simulink model "polytopic_LPV"  (R2020a)
settings: Solver=ode15s  StartTime=0.0  StopTime=10.0  RelTol=1e-3  EnableMultiTasking=on
values from neighbouring files (symbols this model uses):
  p1max = 1/v_min    (= 0.166666666667)    [IPA_polytopes.m]
  p1min = 1/v_max    (= 0.025)    [IPA_polytopes.m]
  p2max = 1/(v_min.*v_min)    [IPA_polytopes.m]
  p2min = 1/(v_max.*v_max)    [IPA_polytopes.m]
  p3max = cos(d_min)    [IPA_polytopes.m]
  p3min = cos(d_max)    [IPA_polytopes.m]
undefined symbols (not defined in the file or in its folder): listK, sigbuilder_block
libraries: cstblocks x19, simulink x2
settings Model: Creator=AHMED  LastModifiedBy=lenovo ideapad
settings DataIOCC: LimitDataPoints=on  SaveFormat=Array  ReturnWorkspaceOutputs=off
settings OptimizationCC: LifeSpan=inf
settings DebuggingCC: SolverPrmCheckMsg=warning  SFUnexpectedBacktrackingDiag=warning  SFNoUnconditionalDefaultTransitionDiag=warning  SFExecutionAtInitializationDiag=none  ArithmeticOperatorsInVariantConditions=warning
settings HardwareCC: ProdBitPerPointer=32  ProdBitPerSizeT=32  ProdBitPerPtrDiffT=32  ProdLargestAtomicFloat=None  ProdIntDivRoundTo=Undefined  ProdEndianess=Unspecified  ProdWordSize=32  ProdHWDeviceType=32-bit Generic
settings ModelReferenceCC: PropagateSignalLabelsOutOfModel=off
settings SFSimCC: SimUseLocalCustomCode=off  CustomCodeUndefinedFunction=UseInterfaceOnly
settings RTWCC: RTWUseLocalCustomCode=off
settings CodeAppCC: StateflowObjectComments=on
settings GRTTargetCC: TargetLangStandard=C89/C90 (ANSI)
settings ConfigComp: CovMetricSettings=dw  CovHtmlReporting=on  CovSaveCumulativeToWorkspaceVar=on  CovSaveSingleToWorkspaceVar=on  CovExternalEMLEnable=off  CovSFcnEnable=off

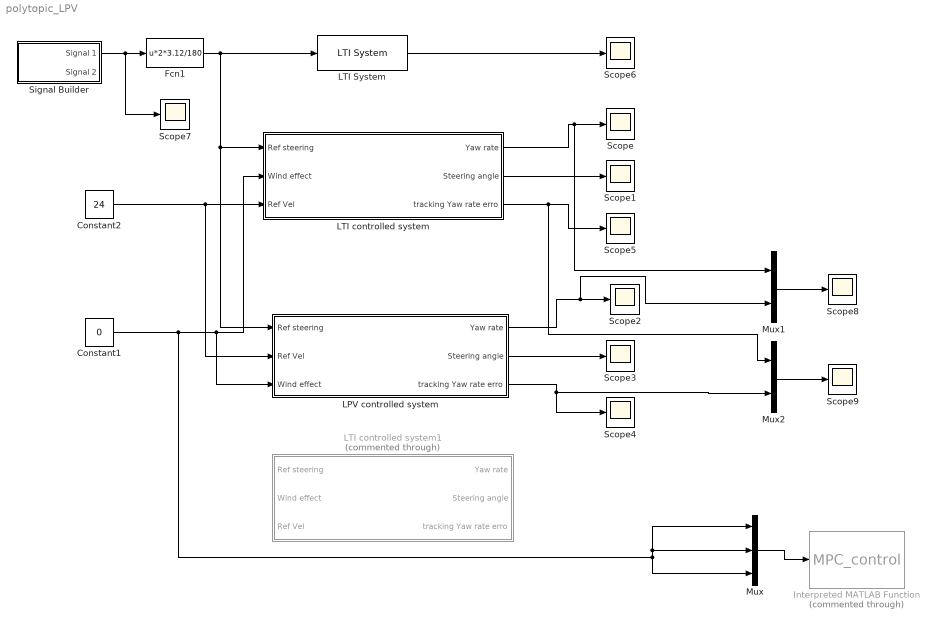
== system polytopic_LPV ==
  Constant1 : Constant  Value=0
  Constant2 : Constant  Value=24
  Fcn1 : Fcn  Expr=u*2*3.12/180
  Interpreted MATLAB Function : MATLABFcn  Commented=through  MATLABFcn=MPC_control  OutputDimensions=3
  LPV controlled system : Subsystem
  LTI System : cstblocks/LTI System  sys=Pr  IC=[]
  LTI controlled system : Subsystem
  LTI controlled system1 : Subsystem  Commented=through
  Mux : Mux  Inputs=3
  Mux1 : Mux  Inputs=2
  Mux2 : Mux  Inputs=2
  Scope{,1..9} (10 alike) : Scope
  Signal Builder : Subsystem  Tag=STV Subsys  LoadFcn=sigbuilder_block('load');  StartFcn=sigbuilder_block('start');  StopFcn=sigbuilder_block('stop');  ClipboardFcn=sigbuilder_block('clipboard');  mask(Sigbuilder block){tuvar=[0:10]}
      mask help: Simulink:masks:SigbuilderBlock_MD
      mask init:
      | if ~strcmp(get_param(bdroot(gcbh),'SimulationStatus'),'stopped') tuvar = sigbuilder_block('maskInit'); end
      settings: CopyFcn=sigbuilder_block('copy');  DeleteFcn=sigbuilder_block('delete');  ModelCloseFcn=sigbuilder_block('modelClose');  PreSaveFcn=sigbuilder_block('preSave');  PauseFcn=sigbuilder_block('pause');  ContinueFcn=sigbuilder_block('continue');  NameChangeFcn=sigbuilder_block('namechange');  OpenFcn=sigbuilder_block('open',[6 28.5 1012.5 483.75 ]);  CloseFcn=sigbuilder_block('close');
      mask Display: plot(0, 0, 100, 100,[2, 2, 32, 32, 2], [68, 8, 8, 68, 68],[32, 2], [38, 38], [32, 19, 2],[53, 60, 44], [32, 17, 17, 2],[16, 16, 31, 31]);txt = getActiveGroup(gcbh);text(2, 100, txt,'verticalAlignment', 'top');
  wires:
  LTI controlled system/1(Yaw rate) -> Mux1/1, Scope/1
  LTI controlled system/2(Steering angle) -> Scope1/1
  LPV controlled system/1(Yaw rate) -> Mux1/2, Scope2/1
  LPV controlled system/2(Steering angle) -> Scope3/1
  Constant2/1 -> LPV controlled system/2(Ref Vel), LTI controlled system/3(Ref Vel)
  Constant1/1 -> Mux/2, Mux/1, Mux/3, LPV controlled system/3(Wind effect), LTI controlled system/2(Wind effect)
  Fcn1/1 -> LTI System/1, LPV controlled system/1(Ref steering), LTI controlled system/1(Ref steering)
  LTI System/1 -> Scope6/1
  Mux/1 -> Interpreted MATLAB Function/1
  Signal Builder/1(Signal 1) -> Scope7/1, Fcn1/1
  Mux1/1 -> Scope8/1
  LTI controlled system/3(tracking Yaw rate erro) -> Mux2/1, Scope5/1
  LPV controlled system/3(tracking Yaw rate erro) -> Mux2/2, Scope4/1
  Mux2/1 -> Scope9/1

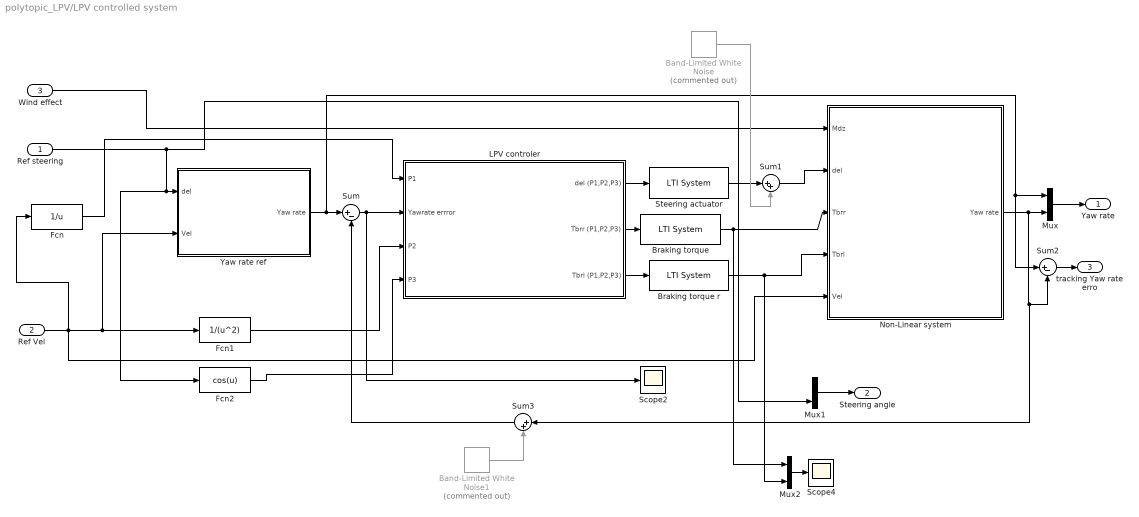
== system polytopic_LPV/LPV controlled system ==
  Ref steering : Inport
  Ref Vel : Inport  Port=2
  Wind effect : Inport  Port=3
  Band-Limited White Noise : simulink/Sources/Band-Limited White Noise  Commented=on  Cov=[0.1]  Ts=0.1  seed=[23341]
  Band-Limited White Noise1 : simulink/Sources/Band-Limited White Noise  Commented=on  Cov=[0.1]  Ts=0.1  seed=[23341]
  Braking torque : cstblocks/LTI System  sys=WactBr  IC=[]
  Braking torque r : cstblocks/LTI System  sys=WactBl  IC=[]
  Fcn : Fcn  Expr=1/u
  Fcn1 : Fcn  Expr=1/(u^2)
  Fcn2 : Fcn  Expr=cos(u)
  LPV controler : Subsystem
  Mux : Mux  Inputs=2
  Mux1 : Mux  Inputs=2
  Mux2 : Mux  Inputs=2
  Non-Linear system : Subsystem
  Scope2 : Scope
  Scope4 : Scope
  Steering actuator : cstblocks/LTI System  sys=WactS  IC=[]
  Sum : Sum  Inputs=|+-
  Sum1 : Sum  Inputs=|++
  Sum2 : Sum  Inputs=|+-
  Sum3 : Sum  Inputs=|++
  Yaw rate ref : Subsystem
  Yaw rate : Outport
  Steering angle : Outport  Port=2
  tracking Yaw rate erro : Outport  Port=3
  wires:
  Sum/1 -> LPV controler/2("Yawrate errror "), Scope2/1
  Wind effect/1 -> Non-Linear system/1(Mdz)
  Ref Vel/1 -> Non-Linear system/5(Vel), Yaw rate ref/2(Vel), Fcn1/1, Fcn/1
  Ref steering/1 -> Mux1/2, Yaw rate ref/1(del), Fcn2/1
  Mux/1 -> Yaw rate/1
  Mux2/1 -> Scope4/1
  Mux1/1 -> Steering angle/1
  Fcn2/1 -> LPV controler/4(P3)
  LPV controler/1(del (P1,P2,P3)) -> Steering actuator/1
  LPV controler/3(Tbrl (P1,P2,P3)) -> Braking torque r/1
  LPV controler/2(Tbrr (P1,P2,P3)) -> Braking torque/1
  Fcn/1 -> LPV controler/1(P1)
  Fcn1/1 -> LPV controler/3(P2)
  Yaw rate ref/1(Yaw rate) -> Sum/1, Sum2/1, Mux/1
  Non-Linear system/1(Yaw rate) -> Sum3/1, Sum2/2, Mux/2
  Sum2/1 -> tracking Yaw rate erro/1
  Braking torque/1 -> Mux2/1, Non-Linear system/3(Tbrr)
  Braking torque r/1 -> Mux2/2, Non-Linear system/4(Tbrl)
  Steering actuator/1 -> Sum1/1
  Band-Limited White Noise/1 -> Sum1/2
  Sum1/1 -> Non-Linear system/2(del)
  Sum3/1 -> Sum/2
  Band-Limited White Noise1/1 -> Sum3/2

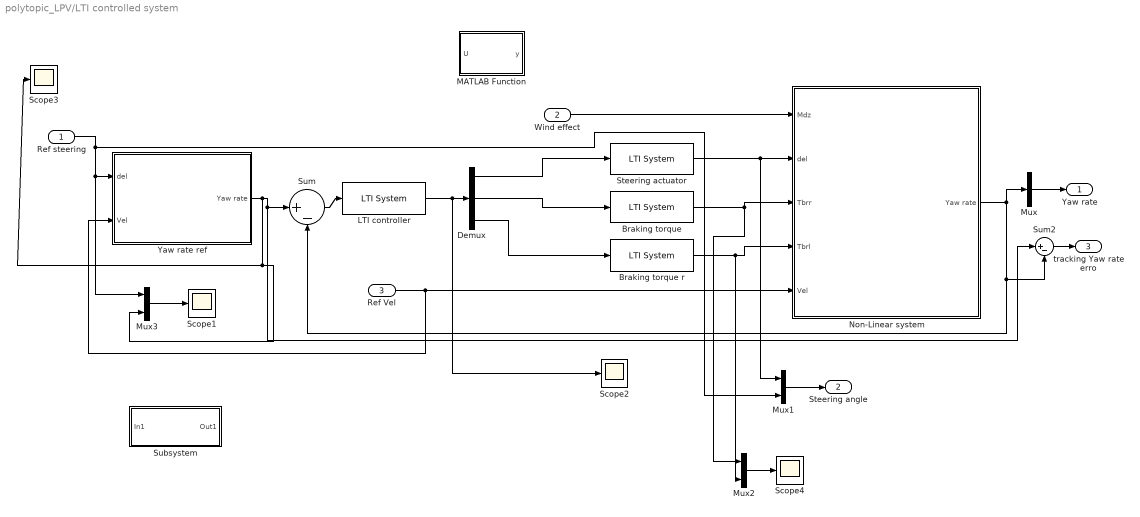
== system polytopic_LPV/LTI controlled system ==
  Ref steering : Inport
  Wind effect : Inport  Port=2
  Ref Vel : Inport  Port=3
  Braking torque : cstblocks/LTI System  sys=WactBr  IC=[]
  Braking torque r : cstblocks/LTI System  sys=WactBl  IC=[]
  Demux : Demux  Outputs=3
  LTI controller : cstblocks/LTI System  sys=KLTI  IC=[]
  MATLAB Function : MATLAB Function  TreatAsAtomicUnit=on
  Mux : Mux  Inputs=1
  Mux1 : Mux  Inputs=2
  Mux2 : Mux  Inputs=2
  Mux3 : Mux  Inputs=2
  Non-Linear system : Subsystem
  Scope{1..4} (4 alike) : Scope
  Steering actuator : cstblocks/LTI System  sys=WactS  IC=[]
  Subsystem : Subsystem
  Sum : Sum  Inputs=|+-
  Sum2 : Sum  Inputs=|+-
  Yaw rate ref : Subsystem
  Yaw rate : Outport
  Steering angle : Outport  Port=2
  tracking Yaw rate erro : Outport  Port=3
  wires:
  Yaw rate ref/1(Yaw rate) -> Sum2/1, Sum/1, Mux3/2, Scope3/1
  Sum/1 -> LTI controller/1
  LTI controller/1 -> Scope2/1, Demux/1
  Non-Linear system/1(Yaw rate) -> Mux/1, Sum2/2, Sum/2
  Wind effect/1 -> Non-Linear system/1(Mdz)
  Ref Vel/1 -> Yaw rate ref/2(Vel), Non-Linear system/5(Vel)
  Ref steering/1 -> Mux1/2, Yaw rate ref/1(del), Mux3/1
  Mux/1 -> Yaw rate/1
  Demux/1 -> Steering actuator/1
  Braking torque r/1 -> Mux2/2, Non-Linear system/4(Tbrl)
  Demux/3 -> Braking torque r/1
  Steering actuator/1 -> Non-Linear system/2(del), Mux1/1
  Demux/2 -> Braking torque/1
  Braking torque/1 -> Mux2/1, Non-Linear system/3(Tbrr)
  Mux2/1 -> Scope4/1
  Mux1/1 -> Steering angle/1
  Mux3/1 -> Scope1/1
  Sum2/1 -> tracking Yaw rate erro/1

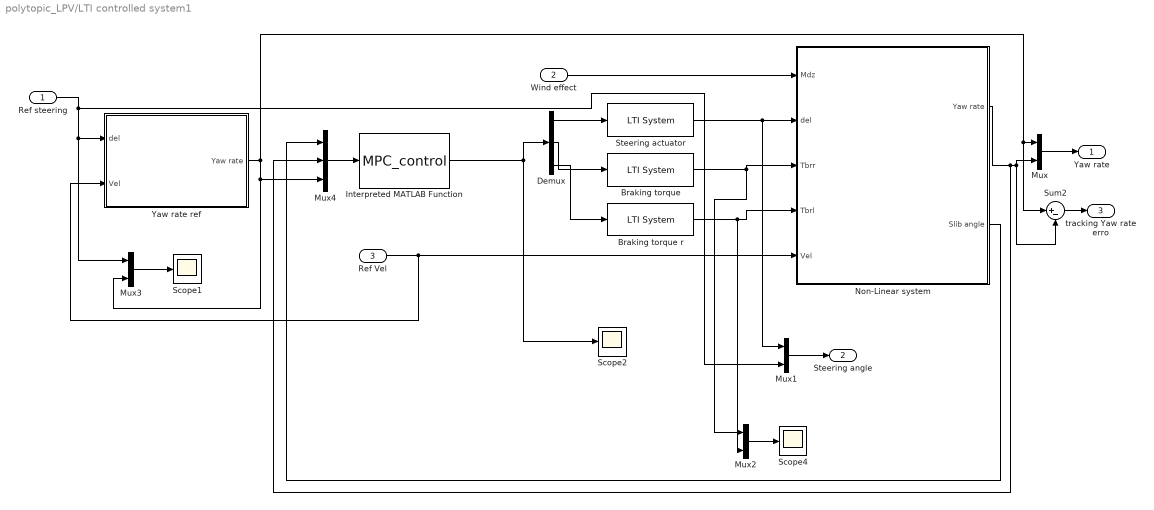
== system polytopic_LPV/LTI controlled system1 ==
  Ref steering : Inport
  Wind effect : Inport  Port=2
  Ref Vel : Inport  Port=3
  Braking torque : cstblocks/LTI System  sys=WactBr  IC=[]
  Braking torque r : cstblocks/LTI System  sys=WactBl  IC=[]
  Demux : Demux  Outputs=3
  Interpreted MATLAB Function : MATLABFcn  MATLABFcn=MPC_control  OutputDimensions=3
  Mux{,1..3} (4 alike) : Mux  Inputs=2
  Mux4 : Mux  Inputs=3
  Non-Linear system : Subsystem
  Scope1 : Scope
  Scope2 : Scope
  Scope4 : Scope
  Steering actuator : cstblocks/LTI System  sys=WactS  IC=[]
  Sum2 : Sum  Inputs=|+-
  Yaw rate ref : Subsystem
  Yaw rate : Outport
  Steering angle : Outport  Port=2
  tracking Yaw rate erro : Outport  Port=3
  wires:
  Yaw rate ref/1(Yaw rate) -> Mux4/3, Mux3/2, Sum2/1, Mux/1
  Interpreted MATLAB Function/1 -> Scope2/1, Demux/1
  Non-Linear system/1(Yaw rate) -> Mux4/2, Sum2/2, Mux/2
  Wind effect/1 -> Non-Linear system/1(Mdz)
  Ref Vel/1 -> Yaw rate ref/2(Vel), Non-Linear system/5(Vel)
  Ref steering/1 -> Mux1/2, Yaw rate ref/1(del), Mux3/1
  Mux/1 -> Yaw rate/1
  Demux/1 -> Steering actuator/1
  Braking torque r/1 -> Mux2/2, Non-Linear system/4(Tbrl)
  Demux/3 -> Braking torque r/1
  Steering actuator/1 -> Non-Linear system/2(del), Mux1/1
  Demux/2 -> Braking torque/1
  Braking torque/1 -> Mux2/1, Non-Linear system/3(Tbrr)
  Mux2/1 -> Scope4/1
  Mux1/1 -> Steering angle/1
  Mux3/1 -> Scope1/1
  Sum2/1 -> tracking Yaw rate erro/1
  Mux4/1 -> Interpreted MATLAB Function/1
  Non-Linear system/2(Slib angle) -> Mux4/1

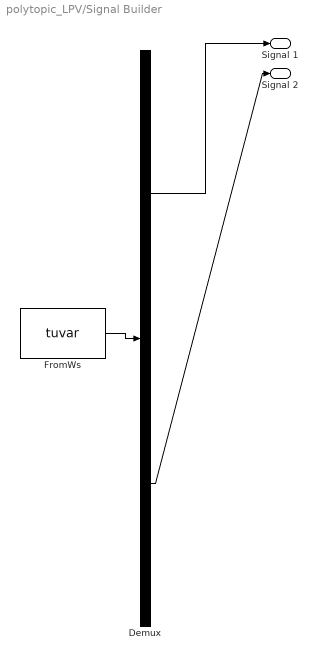
== system polytopic_LPV/Signal Builder ==
  Demux : Demux  Tag=STV Demux  Outputs=2
      settings: DisplayOption=none
  FromWs : FromWorkspace  Tag=STV FromWs  VariableName=tuvar
      SigBuilderData=|
      | common.afterFinalStr = 'Extrapolate'
      | common.sampleTime = 0
      | dataSet.timeRange = [0 10]
      | dataSet.name = 'Group 1'
      | sbobj.Groups.Name = 'Group 1'
      | sbobj.Groups.Signals(1).Name = 'Signal 1'
      | sbobj.Groups.Signals(1).XData = [0 0.98 2 2 3.02 3.02 4.96 4.96 6.04 6.04 6.98 10]
      | sbobj.Groups.Signals(1).YData = [0 0 10 9.95 9.95 10.05 -10 -10.05 -10.05 -9.9 -0.02 0]
      | sbobj.Groups.Signals(2).Name = 'Signal 2'
      | sbobj.Groups.Signals(2).XData = [0 2.04 2.04 2.58 2.58 4.94 4.94 6.98 10]
      | sbobj.Groups.Signals(2).YData = [0 0 0.01 11.2 11.3 11.3 11.4 0 0]
  Signal 1 : Outport  Tag=STV Outport
  Signal 2 : Outport  Tag=STV Outport  Port=2
  wires:
  Demux/1 -> Signal 1/1
  FromWs/1 -> Demux/1
  Demux/2 -> Signal 2/1

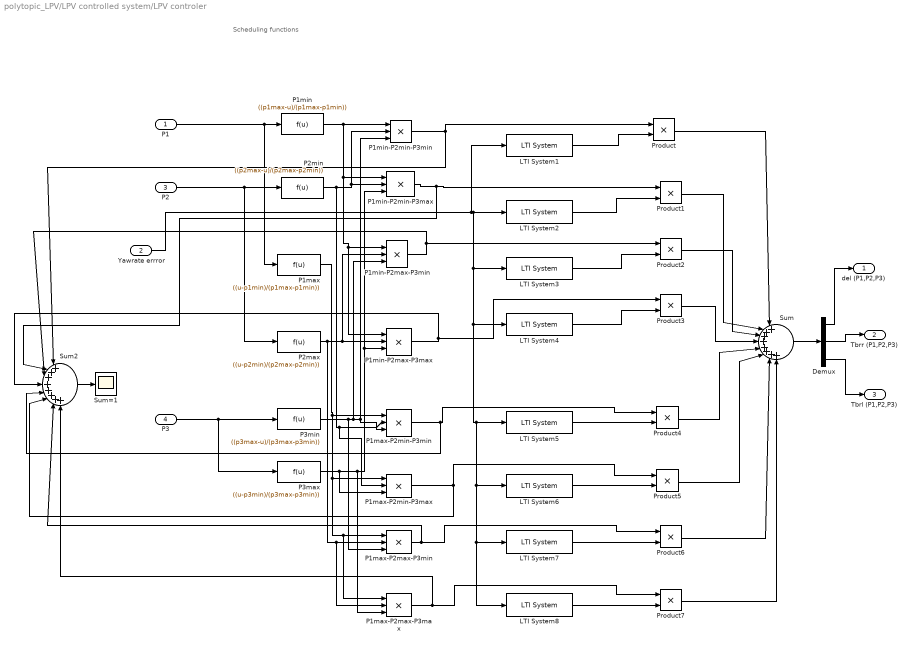
== system polytopic_LPV/LPV controlled system/LPV controler ==
  note: Scheduling functions
  P1 : Inport
  "Yawrate errror " : Inport  Port=2
  P2 : Inport  Port=3
  P3 : Inport  Port=4
  Demux : Demux  Outputs=3
  LTI System1 : cstblocks/LTI System  sys=listK{1}  IC=[]
  LTI System2 : cstblocks/LTI System  sys=listK{2}  IC=[]
  LTI System3 : cstblocks/LTI System  sys=listK{3}  IC=[]
  LTI System4 : cstblocks/LTI System  sys=listK{4}  IC=[]
  LTI System5 : cstblocks/LTI System  sys=listK{5}  IC=[]
  LTI System6 : cstblocks/LTI System  sys=listK{6}  IC=[]
  LTI System7 : cstblocks/LTI System  sys=listK{7}  IC=[]
  LTI System8 : cstblocks/LTI System  sys=listK{8}  IC=[]
  P1max : Fcn  Expr=((u-p1min)/(p1max-p1min))
  P1max-P2max-P3max : Product  Inputs=3
  P1max-P2max-P3min : Product  Inputs=3
  P1max-P2min-P3max : Product  Inputs=3
  P1max-P2min-P3min : Product  Inputs=3
  P1min : Fcn  Expr=((p1max-u)/(p1max-p1min))
  P1min-P2max-P3max : Product  Inputs=3
  P1min-P2max-P3min : Product  Inputs=3
  P1min-P2min-P3max : Product  Inputs=3
  P1min-P2min-P3min : Product  Inputs=3
  P2max : Fcn  Expr=((u-p2min)/(p2max-p2min))
  P2min : Fcn  Expr=((p2max-u)/(p2max-p2min))
  P3max : Fcn  Expr=((u-p3min)/(p3max-p3min))
  P3min : Fcn  Expr=((p3max-u)/(p3max-p3min))
  Product{,1..7} (8 alike) : Product
  Sum : Sum  Inputs=|++++++++
  Sum2 : Sum  Inputs=|++++++++
  Sum=1 : Scope
  del (P1,P2,P3) : Outport
  Tbrr (P1,P2,P3) : Outport  Port=2
  Tbrl (P1,P2,P3) : Outport  Port=3
  wires:
  "Yawrate errror "/1 -> LTI System1/1, LTI System8/1, LTI System7/1, LTI System6/1, LTI System5/1, LTI System4/1, LTI System3/1, LTI System2/1
  LTI System1/1 -> Product/2
  P1min-P2min-P3min/1 -> Product/1, Sum2/1
  P1min-P2min-P3max/1 -> Sum2/2, Product1/1
  LTI System2/1 -> Product1/2
  P1min-P2max-P3min/1 -> Product2/1, Sum2/3
  LTI System3/1 -> Product2/2
  P1min-P2max-P3max/1 -> Product3/1, Sum2/4
  LTI System4/1 -> Product3/2
  Product/1 -> Sum/1
  Product1/1 -> Sum/2
  Product2/1 -> Sum/3
  Product3/1 -> Sum/4
  P2max/1 -> P1max-P2max-P3max/2, P1max-P2max-P3min/2, P1min-P2max-P3min/2, P1min-P2max-P3max/2
  P2min/1 -> P1max-P2min-P3max/2, P1max-P2min-P3min/2, P1min-P2min-P3max/2, P1min-P2min-P3min/2
  P1min/1 -> P1min-P2max-P3max/1, P1min-P2max-P3min/1, P1min-P2min-P3max/1, P1min-P2min-P3min/1
  P1/1 -> P1max/1, P1min/1
  P2/1 -> P2max/1, P2min/1
  Sum2/1 -> Sum=1/1
  P3/1 -> P3max/1, P3min/1
  P3min/1 -> P1max-P2max-P3min/3, P1min-P2max-P3min/3, P1min-P2min-P3min/3, P1max-P2min-P3min/3
  P3max/1 -> P1max-P2min-P3max/3, P1min-P2min-P3max/3, P1min-P2max-P3max/3, P1max-P2max-P3max/3
  P1max/1 -> P1max-P2max-P3max/1, P1max-P2max-P3min/1, P1max-P2min-P3max/1, P1max-P2min-P3min/1
  LTI System5/1 -> Product4/2
  LTI System6/1 -> Product5/2
  LTI System7/1 -> Product6/2
  LTI System8/1 -> Product7/2
  P1max-P2min-P3min/1 -> Sum2/5, Product4/1
  P1max-P2min-P3max/1 -> Product5/1, Sum2/6
  P1max-P2max-P3min/1 -> Product6/1, Sum2/7
  P1max-P2max-P3max/1 -> Product7/1, Sum2/8
  Product4/1 -> Sum/5
  Product5/1 -> Sum/6
  Product6/1 -> Sum/7
  Product7/1 -> Sum/8
  Sum/1 -> Demux/1
  Demux/1 -> del (P1,P2,P3)/1
  Demux/2 -> Tbrr (P1,P2,P3)/1
  Demux/3 -> Tbrl (P1,P2,P3)/1

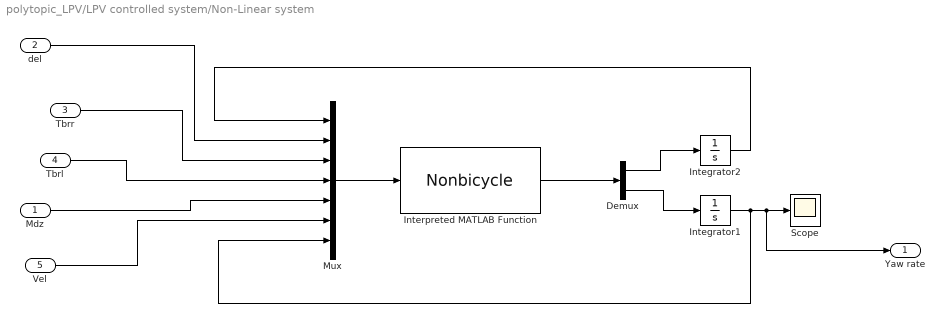
== system polytopic_LPV/LPV controlled system/Non-Linear system ==
  Mdz : Inport
  del : Inport  Port=2
  Tbrr : Inport  Port=3
  Tbrl : Inport  Port=4
  Vel : Inport  Port=5
  Demux : Demux  Outputs=2
  Integrator1 : Integrator
  Integrator2 : Integrator
  Interpreted MATLAB Function : MATLABFcn  MATLABFcn=Nonbicycle  OutputDimensions=2
  Mux : Mux  Inputs=7
  Scope : Scope
  Yaw rate : Outport
  wires:
  Mux/1 -> Interpreted MATLAB Function/1
  Interpreted MATLAB Function/1 -> Demux/1
  Demux/1 -> Integrator2/1
  Demux/2 -> Integrator1/1
  Integrator2/1 -> Mux/1
  Integrator1/1 -> Yaw rate/1, Scope/1, Mux/7
  del/1 -> Mux/2
  Vel/1 -> Mux/6
  Tbrr/1 -> Mux/3
  Tbrl/1 -> Mux/4
  Mdz/1 -> Mux/5

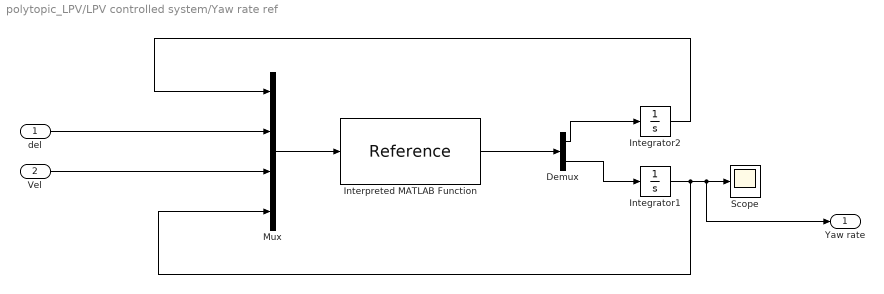
== system polytopic_LPV/LPV controlled system/Yaw rate ref ==
  del : Inport
  Vel : Inport  Port=2
  Demux : Demux  Outputs=2
  Integrator1 : Integrator
  Integrator2 : Integrator
  Interpreted MATLAB Function : MATLABFcn  MATLABFcn=Reference  OutputDimensions=2
  Mux : Mux
  Scope : Scope
  Yaw rate : Outport
  wires:
  Mux/1 -> Interpreted MATLAB Function/1
  Interpreted MATLAB Function/1 -> Demux/1
  Demux/1 -> Integrator2/1
  Demux/2 -> Integrator1/1
  Integrator2/1 -> Mux/1
  Integrator1/1 -> Mux/4, Yaw rate/1, Scope/1
  del/1 -> Mux/2
  Vel/1 -> Mux/3

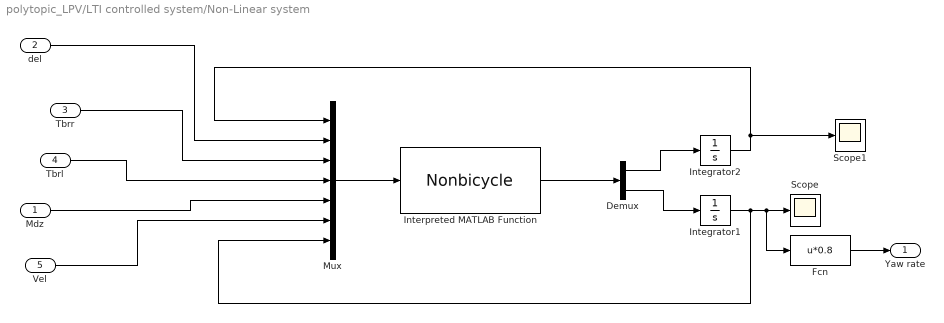
== system polytopic_LPV/LTI controlled system/Non-Linear system ==
  Mdz : Inport
  del : Inport  Port=2
  Tbrr : Inport  Port=3
  Tbrl : Inport  Port=4
  Vel : Inport  Port=5
  Demux : Demux  Outputs=2
  Fcn : Fcn  Expr=u*0.8
  Integrator1 : Integrator
  Integrator2 : Integrator
  Interpreted MATLAB Function : MATLABFcn  MATLABFcn=Nonbicycle  OutputDimensions=2
  Mux : Mux  Inputs=7
  Scope : Scope
  Scope1 : Scope
  Yaw rate : Outport
  wires:
  Mux/1 -> Interpreted MATLAB Function/1
  Interpreted MATLAB Function/1 -> Demux/1
  Demux/1 -> Integrator2/1
  Demux/2 -> Integrator1/1
  Integrator2/1 -> Scope1/1, Mux/1
  Integrator1/1 -> Fcn/1, Scope/1, Mux/7
  del/1 -> Mux/2
  Vel/1 -> Mux/6
  Tbrr/1 -> Mux/3
  Tbrl/1 -> Mux/4
  Mdz/1 -> Mux/5
  Fcn/1 -> Yaw rate/1

== system polytopic_LPV/LTI controlled system/Subsystem ==
  In1 : Inport
  Out1 : Outport
  wires:
  In1/1 -> Out1/1

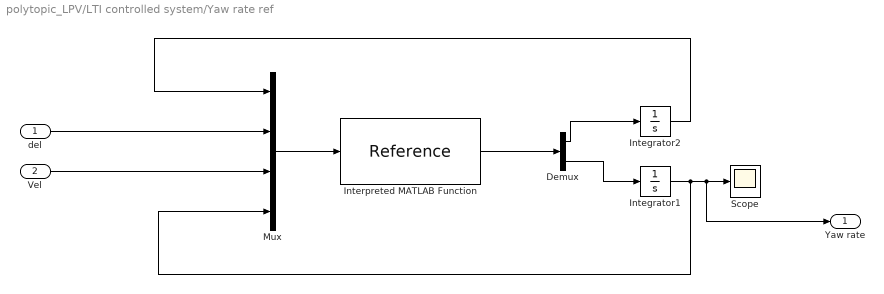
== system polytopic_LPV/LTI controlled system/Yaw rate ref ==
  del : Inport
  Vel : Inport  Port=2
  Demux : Demux  Outputs=2
  Integrator1 : Integrator
  Integrator2 : Integrator
  Interpreted MATLAB Function : MATLABFcn  MATLABFcn=Reference  OutputDimensions=2
  Mux : Mux
  Scope : Scope
  Yaw rate : Outport
  wires:
  Mux/1 -> Interpreted MATLAB Function/1
  Interpreted MATLAB Function/1 -> Demux/1
  Demux/1 -> Integrator2/1
  Demux/2 -> Integrator1/1
  Integrator2/1 -> Mux/1
  Integrator1/1 -> Mux/4, Yaw rate/1, Scope/1
  del/1 -> Mux/2
  Vel/1 -> Mux/3

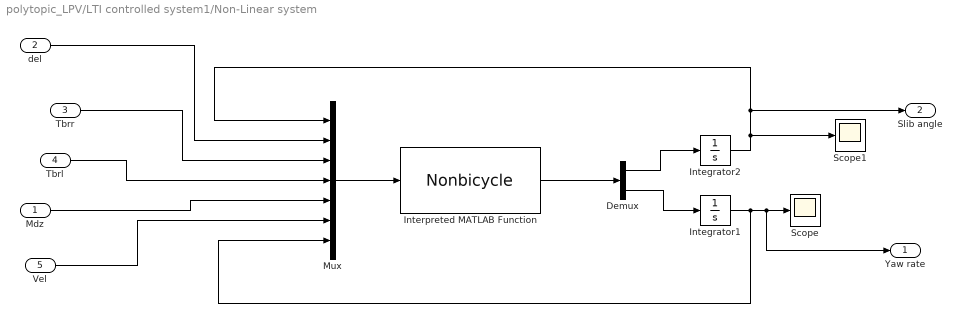
== system polytopic_LPV/LTI controlled system1/Non-Linear system ==
  Mdz : Inport
  del : Inport  Port=2
  Tbrr : Inport  Port=3
  Tbrl : Inport  Port=4
  Vel : Inport  Port=5
  Demux : Demux  Outputs=2
  Integrator1 : Integrator
  Integrator2 : Integrator
  Interpreted MATLAB Function : MATLABFcn  MATLABFcn=Nonbicycle  OutputDimensions=2
  Mux : Mux  Inputs=7
  Scope : Scope
  Scope1 : Scope
  Yaw rate : Outport
  Slib angle : Outport  Port=2
  wires:
  Mux/1 -> Interpreted MATLAB Function/1
  Interpreted MATLAB Function/1 -> Demux/1
  Demux/1 -> Integrator2/1
  Demux/2 -> Integrator1/1
  Integrator2/1 -> Scope1/1, Slib angle/1, Mux/1
  Integrator1/1 -> Yaw rate/1, Scope/1, Mux/7
  del/1 -> Mux/2
  Vel/1 -> Mux/6
  Tbrr/1 -> Mux/3
  Tbrl/1 -> Mux/4
  Mdz/1 -> Mux/5

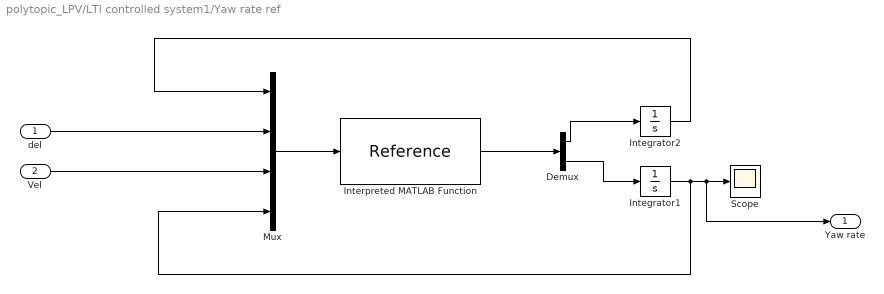
== system polytopic_LPV/LTI controlled system1/Yaw rate ref ==
  del : Inport
  Vel : Inport  Port=2
  Demux : Demux  Outputs=2
  Integrator1 : Integrator
  Integrator2 : Integrator
  Interpreted MATLAB Function : MATLABFcn  MATLABFcn=Reference  OutputDimensions=2
  Mux : Mux
  Scope : Scope
  Yaw rate : Outport
  wires:
  Mux/1 -> Interpreted MATLAB Function/1
  Interpreted MATLAB Function/1 -> Demux/1
  Demux/1 -> Integrator2/1
  Demux/2 -> Integrator1/1
  Integrator2/1 -> Mux/1
  Integrator1/1 -> Mux/4, Yaw rate/1, Scope/1
  del/1 -> Mux/2
  Vel/1 -> Mux/3

== matlab function polytopic_LPV/LTI controlled system/MATLAB Function ==
  data: U input; y output
function y = fcn(U)

parameters

Ur = 1;
beta = U(1);
del = U(2);
Tbrf = U(3);
Tbrr = U(4);
Mdz = U(5);
v = U(6);
psid = U(7);

betadot = (Ur*(-C_f-C_r)/(m*v))*beta + (1+ Ur*(l_r*C_r-l_f*C_f)/(m*v^2))*psid + (C_f/(m*v))*del;
psiddot = (Ur*(l_r*C_r-l_f*C_f*cos(del))/Iz)*beta + (Ur*(-l_f*l_f*C_f*cos(del)-l_r*l_r*C_r)/(Iz*v))*psid + (l_f*C_f*cos(del)/Iz)*del +(1/Iz)*Mdz + (S_rr*R*t_r/2/Iz)*Tbrf - (S_rr*R*t_r/2/Iz)*Tbrr; 

y = [betadot psiddot];
y = u;
